simulink model "our_ch47_rope_load"  (R2020a)
settings: Solver=VariableStepAuto  StartTime=0.0  StopTime=10.0  RelTol=1e-3
undefined symbols (not defined in the file or in its folder): envs, Para_cable, rope1, tandem, trans
settings Model: Creator=tutu  LastModifiedBy=Timo
settings DebuggingCC: InitInArrayFormatMsg=none  SFMachineParentedDataDiag=error

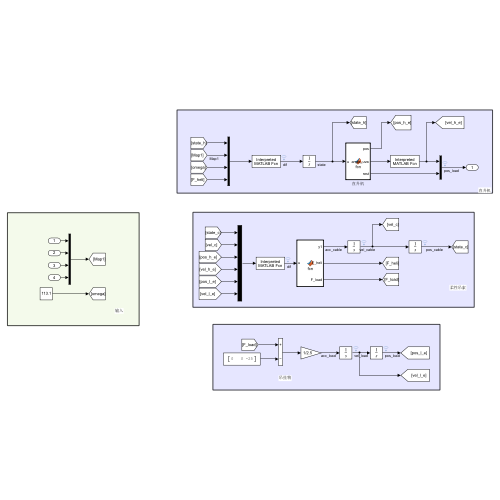
[thumbnail: Simulink's stored preview of the top-level diagram]
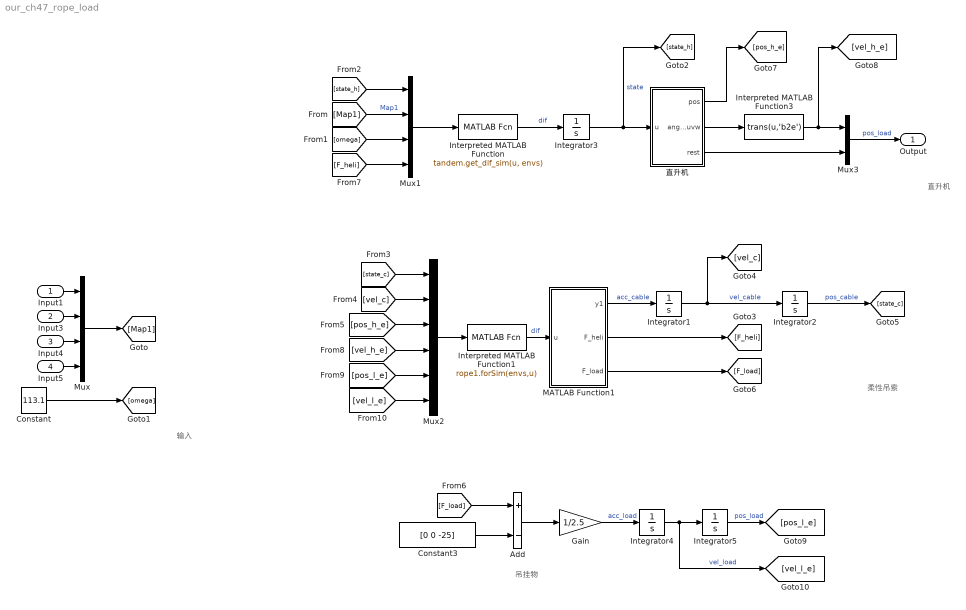
== system our_ch47_rope_load ==
  note: 输入
  note: 吊挂物
  note: 柔性吊索
  note: 直升机
  Input1 : Inport
  Input3 : Inport  Port=2
  Input4 : Inport  Port=3
  Input5 : Inport  Port=4
  Add : Sum  Inputs=+-
  Constant : Constant  Value=113.1
  Constant3 : Constant  Value=[0 0 -25]
  Gain : Gain  Gain=1/2.5
  Integrator1 : Integrator  InitialCondition=zeros(Para_cable.num*3,1)
  Integrator2 : Integrator  InitialCondition=zeros(Para_cable.num*3,1)
  Integrator3 : Integrator
  Integrator4 : Integrator  InitialCondition=zeros(3,1)
  Integrator5 : Integrator  InitialCondition=zeros(3,1)
  Interpreted MATLAB Function : MATLABFcn  MATLABFcn=tandem.get_dif_sim(u, envs)  OutputDimensions=30
  Interpreted MATLAB Function1 : MATLABFcn  MATLABFcn=rope1.forSim(envs,u)  OutputDimensions=Para_cable.num*3+6
  Interpreted MATLAB Function3 : MATLABFcn  MATLABFcn=trans(u,'b2e')  OutputDimensions=3
  MATLAB Function1 : MATLAB Function  TreatAsAtomicUnit=on
  Mux : Mux
  Mux1 : Mux
  Mux2 : Mux  Inputs=6
  Mux3 : Mux  Inputs=2
  直升机 : MATLAB Function  TreatAsAtomicUnit=on
  Output : Outport
  wires:
  Mux/1 -> [Map1]
  Constant/1 -> [omega]
  [state_c] -> Mux2/1
  Integrator4/1 -> [vel_l_e], Integrator5/1  "vel_load"
  Integrator3/1 -> [state_h], 直升机/1(u)  "state"
  Constant3/1 -> Add/2
  MATLAB Function1/2(F_heli) -> [F_heli]
  MATLAB Function1/1(y1) -> Integrator1/1  "acc_cable"
  Integrator1/1 -> Integrator2/1, [vel_c]  "vel_cable"
  Integrator2/1 -> [state_c]  "pos_cable"
  直升机/3(rest) -> Mux3/2
  Mux2/1 -> Interpreted MATLAB Function1/1
  [vel_c] -> Mux2/2
  [vel_l_e] -> Mux2/6
  直升机/2(angle_uvw) -> Interpreted MATLAB Function3/1
  Interpreted MATLAB Function1/1 -> MATLAB Function1/1(u)  "dif"
  Interpreted MATLAB Function/1 -> Integrator3/1  "dif"
  [omega] -> Mux1/3
  [F_load] -> Add/1
  Mux1/1 -> Interpreted MATLAB Function/1
  [state_h] -> Mux1/1
  [Map1] -> Mux1/2  "Map1"
  [pos_h_e] -> Mux2/3
  MATLAB Function1/3(F_load) -> [F_load]
  Gain/1 -> Integrator4/1  "acc_load"
  Add/1 -> Gain/1
  [pos_l_e] -> Mux2/5
  [F_heli] -> Mux1/4
  Integrator5/1 -> [pos_l_e]  "pos_load"
  Input1/1 -> Mux/1
  Input3/1 -> Mux/2
  Input4/1 -> Mux/3
  Input5/1 -> Mux/4
  Mux3/1 -> Output/1  "pos_load"
  直升机/1(pos) -> [pos_h_e]
  Interpreted MATLAB Function3/1 -> [vel_h_e], Mux3/1
  [vel_h_e] -> Mux2/4

== matlab function our_ch47_rope_load/MATLAB Function1 ==
  data: u input; y1 output; F_heli output; F_load output
function [y1, F_heli, F_load] = fcn(u)
num = 10;
y1 = u(1:num*3);
F_heli = u(num*3+1:num*3+3);
F_load = u(num*3+4:num*3+6);

== matlab function our_ch47_rope_load/直升机 ==
  data: pos output; u input; angle_uvw output; rest output
function [pos, angle_uvw, rest]   = fcn(u)
pos = u(10:12);
angle_uvw = [rad2deg(u(7:9)); u(1:3)];
rest = u(4:size(u,1));
end
